simulink model "openloop"  (R2018a)
settings: Solver=VariableStepAuto  StartTime=0.0  StopTime=1  FixedStep=Ts  RelTol=1e-3
values from neighbouring files (symbols this model uses):
  A = [cos(theta) -sin(theta) 0 0;sin(theta) cos(theta) 0 0;0 0 1 0;0 0 0 1]*     [1 0 0 0; 0 1 0 0; 0 0 1 d; 0 0 0 1]*     [1 0 0 a; 0 1 0 0; 0 0 1 0; 0 0 0 1]*     [1 0 0 0; 0 0 1 0;0 -1 0 0;0 0 0 1]    [DE_Generator.m]    (also in GUI_ellipsoid.m = [0 1; 0 0]; question3.m = double(subs(DziDzj)); question4.m = [])
  B = [0; 1]    [GUI_ellipsoid.m]    (also in question3.m = double(subs(DziDuj)); question4.m)
  Ts = 0.01    [GUI_ellipsoid.m]    (also in question3.m; question4.m)
  z0 = zb*1.2    [question3.m]
undefined symbols (not defined in the file or in its folder): Ak, Bk, stateder
settings Model: Creator=rhanz  LastModifiedBy=erivelton

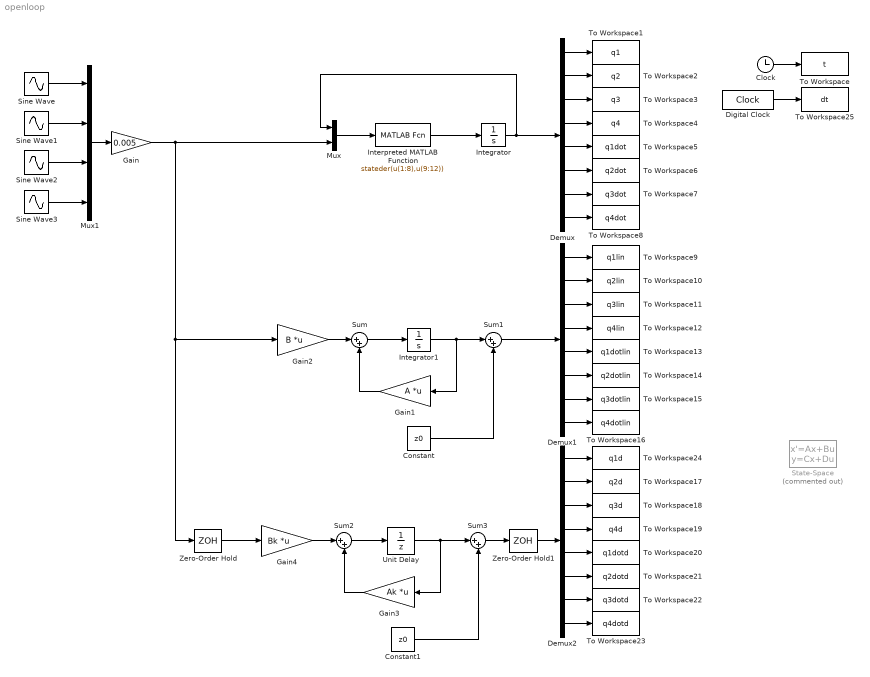
== system openloop ==
  Clock : Clock
  Constant : Constant  Value=z0
  Constant1 : Constant  Value=z0
  Demux : Demux  Outputs=8
  Demux1 : Demux  Outputs=8
  Demux2 : Demux  Outputs=8
  Digital Clock : DigitalClock  SampleTime=Ts
  Gain : Gain  Gain=0.005
  Gain1 : Gain  Gain=A  Multiplication=Matrix(K*u) (u vector)
  Gain2 : Gain  Gain=B  Multiplication=Matrix(K*u) (u vector)
  Gain3 : Gain  Gain=Ak  Multiplication=Matrix(K*u) (u vector)
  Gain4 : Gain  Gain=Bk  Multiplication=Matrix(K*u) (u vector)
  Integrator : Integrator  InitialCondition=z0
  Integrator1 : Integrator
  Interpreted MATLAB Function : MATLABFcn  MATLABFcn=stateder(u(1:8),u(9:12))  OutputDimensions=8
  Mux : Mux  Inputs=2
  Mux1 : Mux
  Sine Wave{,1..3} (4 alike) : Sin  Frequency=5  SampleTime=0
  State-Space : StateSpace  Commented=on  A=A  B=B  C=eye(8)  D=zeros(8,4)  InitialCondition=0
  Sum{,1..3} (4 alike) : Sum  Inputs=|++
  To Workspace : ToWorkspace  VariableName=t  SampleTime=-1
  To Workspace1 : ToWorkspace  VariableName=q1  SampleTime=-1
  To Workspace10 : ToWorkspace  VariableName=q2lin  SampleTime=-1
  To Workspace11 : ToWorkspace  VariableName=q3lin  SampleTime=-1
  To Workspace12 : ToWorkspace  VariableName=q4lin  SampleTime=-1
  To Workspace13 : ToWorkspace  VariableName=q1dotlin  SampleTime=-1
  To Workspace14 : ToWorkspace  VariableName=q2dotlin  SampleTime=-1
  To Workspace15 : ToWorkspace  VariableName=q3dotlin  SampleTime=-1
  To Workspace16 : ToWorkspace  VariableName=q4dotlin  SampleTime=-1
  To Workspace17 : ToWorkspace  VariableName=q2d  SampleTime=-1
  To Workspace18 : ToWorkspace  VariableName=q3d  SampleTime=-1
  To Workspace19 : ToWorkspace  VariableName=q4d  SampleTime=-1
  To Workspace2 : ToWorkspace  VariableName=q2  SampleTime=-1
  To Workspace20 : ToWorkspace  VariableName=q1dotd  SampleTime=-1
  To Workspace21 : ToWorkspace  VariableName=q2dotd  SampleTime=-1
  To Workspace22 : ToWorkspace  VariableName=q3dotd  SampleTime=-1
  To Workspace23 : ToWorkspace  VariableName=q4dotd  SampleTime=-1
  To Workspace24 : ToWorkspace  VariableName=q1d  SampleTime=-1
  To Workspace25 : ToWorkspace  VariableName=dt  SampleTime=-1
  To Workspace3 : ToWorkspace  VariableName=q3  SampleTime=-1
  To Workspace4 : ToWorkspace  VariableName=q4  SampleTime=-1
  To Workspace5 : ToWorkspace  VariableName=q1dot  SampleTime=-1
  To Workspace6 : ToWorkspace  VariableName=q2dot  SampleTime=-1
  To Workspace7 : ToWorkspace  VariableName=q3dot  SampleTime=-1
  To Workspace8 : ToWorkspace  VariableName=q4dot  SampleTime=-1
  To Workspace9 : ToWorkspace  VariableName=q1lin  SampleTime=-1
  Unit Delay : UnitDelay  SampleTime=-1
  Zero-Order Hold : ZeroOrderHold  SampleTime=Ts
  Zero-Order Hold1 : ZeroOrderHold  SampleTime=Ts
  wires:
  Interpreted MATLAB Function/1 -> Integrator/1
  Mux/1 -> Interpreted MATLAB Function/1
  Integrator/1 -> Mux/1, Demux/1
  Sine Wave1/1 -> Mux1/2
  Sine Wave2/1 -> Mux1/3
  Sine Wave3/1 -> Mux1/4
  Sine Wave/1 -> Mux1/1
  Mux1/1 -> Gain/1
  Clock/1 -> To Workspace/1
  Demux/1 -> To Workspace1/1
  Demux/2 -> To Workspace2/1
  Demux/3 -> To Workspace3/1
  Demux/4 -> To Workspace4/1
  Demux/5 -> To Workspace5/1
  Demux/6 -> To Workspace6/1
  Demux/7 -> To Workspace7/1
  Demux/8 -> To Workspace8/1
  Sum/1 -> Integrator1/1
  Gain1/1 -> Sum/2
  Gain2/1 -> Sum/1
  Integrator1/1 -> Sum1/1, Gain1/1
  Constant/1 -> Sum1/2
  Demux1/6 -> To Workspace14/1
  Demux1/5 -> To Workspace13/1
  Demux1/4 -> To Workspace12/1
  Demux1/3 -> To Workspace11/1
  Demux1/2 -> To Workspace10/1
  Demux1/1 -> To Workspace9/1
  Sum1/1 -> Demux1/1
  Demux1/7 -> To Workspace15/1
  Demux1/8 -> To Workspace16/1
  Gain/1 -> Mux/2, Gain2/1, Zero-Order Hold/1
  Zero-Order Hold/1 -> Gain4/1
  Sum3/1 -> Zero-Order Hold1/1
  Demux2/2 -> To Workspace17/1
  Demux2/4 -> To Workspace19/1
  Zero-Order Hold1/1 -> Demux2/1
  Demux2/7 -> To Workspace22/1
  Demux2/1 -> To Workspace24/1
  Demux2/8 -> To Workspace23/1
  Demux2/5 -> To Workspace20/1
  Demux2/3 -> To Workspace18/1
  Demux2/6 -> To Workspace21/1
  Digital Clock/1 -> To Workspace25/1
  Unit Delay/1 -> Sum3/1, Gain3/1
  Gain4/1 -> Sum2/1
  Sum2/1 -> Unit Delay/1
  Gain3/1 -> Sum2/2
  Constant1/1 -> Sum3/2
